simulink model "N7_6"  (R2016a)
settings: Solver=VariableStepAuto  StartTime=0.0  StopTime=10.0  RelTol=1e-3
settings Model: Creator=Kayab  LastModifiedBy=Kayab

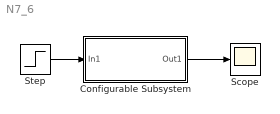
== system N7_6 ==
  Configurable Subsystem : Subsystem  BlockChoice=Transfer Fcn
      settings: AttributesFormatString=%<BlockChoice>  MemberBlocks=Transfer Fcn,Transfer Fcn1
      settings: TemplateBlock=|
      | N7_6lib/Configurable
      | Subsystem
  Scope : Scope
  Step : Step  SampleTime=0
  wires:
  Step/1 -> Configurable Subsystem/1(In1)
  Configurable Subsystem/1(Out1) -> Scope/1

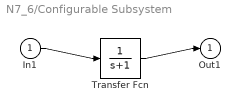
== system N7_6/Configurable Subsystem ==
  In1 : Inport
  Transfer Fcn : TransferFcn  Denominator=[1 1]
  Out1 : Outport
  wires:
  In1/1 -> Transfer Fcn/1
  Transfer Fcn/1 -> Out1/1
